simulink model "Problem3_sim"  (R2018a)
settings: Solver=ode45  StartTime=0.0  StopTime=600  RelTol=1e-3
values from neighbouring files (symbols this model uses):
  g = 9.81    [Problem3.m]
  kd_fi = (2*zeta_fi*omega_fi-alpha_fi1)/alpha_fi2    [Problem3.m]
  ki_chi = omega_chi^2*V_g/g    [Problem3.m]
  ki_fi = -0    (= 0)    [Problem3.m]
  kp_chi = 2*zeta_chi*omega_chi*V_g/g    [Problem3.m]
  kp_fi = -2    [Problem3.m]
  V_g = 580/3.6    (= 161.111111111)    [Problem3.m]
undefined symbols (not defined in the file or in its folder): data
libraries: simulink_extras x2
settings Model: Creator=marti  LastModifiedBy=Anders Vagle
settings OptimizationCC: LifeSpan=inf
settings DebuggingCC: SFExecutionAtInitializationDiag=none
settings HardwareCC: ProdBitPerSizeT=32  ProdBitPerPtrDiffT=32  ProdWordSize=32  ProdHWDeviceType=Specified
settings CodeAppCC: StateflowObjectComments=on

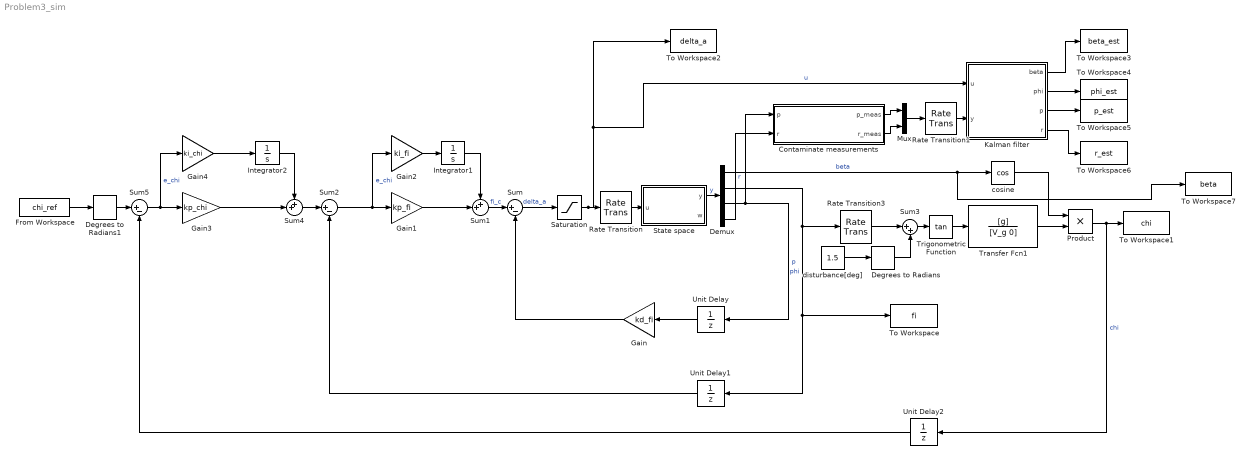
== system Problem3_sim ==
  Contaminate measurements : MATLAB Function  TreatAsAtomicUnit=on
  Degrees to Radians : simulink_extras/Transformations/Degrees to Radians
  Degrees to Radians1 : simulink_extras/Transformations/Degrees to Radians
  Demux : Demux
  From Workspace : FromWorkspace  VariableName=chi_ref  SampleTime=0  Interpolate=off  OutputAfterFinalValue=Holding final value
  Gain : Gain  Gain=kd_fi
  Gain1 : Gain  Gain=kp_fi
  Gain2 : Gain  Gain=ki_fi
  Gain3 : Gain  Gain=kp_chi
  Gain4 : Gain  Gain=ki_chi
  Integrator1 : Integrator
  Integrator2 : Integrator
  Kalman filter : MATLAB Function  TreatAsAtomicUnit=on  mask{data=data}
      mask prompts: data "data struct"
  Mux : Mux  Inputs=2
  Product : Product
  Rate Transition : RateTransition  OutPortSampleTime=Ts
  Rate Transition1 : RateTransition
  Rate Transition3 : RateTransition  OutPortSampleTime=Ts
  Saturation : Saturate  UpperLimit=30/180*pi  LowerLimit=-30/180*pi
  State space : MATLAB Function  TreatAsAtomicUnit=on
  Sum : Sum  Inputs=|+-
  Sum1 : Sum  Inputs=++|
  Sum2 : Sum  Inputs=|+-
  Sum3 : Sum  Inputs=|++
  Sum4 : Sum  Inputs=++|
  Sum5 : Sum  Inputs=|+-
  To Workspace : ToWorkspace  VariableName=fi  SaveFormat=Timeseries  SampleTime=-1
  To Workspace1 : ToWorkspace  VariableName=chi  SaveFormat=Timeseries  SampleTime=-1
  To Workspace2 : ToWorkspace  VariableName=delta_a  SaveFormat=Timeseries  SampleTime=-1
  To Workspace3 : ToWorkspace  VariableName=beta_est  SaveFormat=Timeseries  SampleTime=-1
  To Workspace4 : ToWorkspace  VariableName=phi_est  SaveFormat=Timeseries  SampleTime=-1
  To Workspace5 : ToWorkspace  VariableName=p_est  SaveFormat=Timeseries  SampleTime=-1
  To Workspace6 : ToWorkspace  VariableName=r_est  SaveFormat=Timeseries  SampleTime=-1
  To Workspace7 : ToWorkspace  VariableName=beta  SaveFormat=Timeseries  SampleTime=-1
  Transfer Fcn1 : TransferFcn  Numerator=[g]  Denominator=[V_g 0]
  Trigonometric Function : Trigonometry  Operator=tan
  Unit Delay : UnitDelay  SampleTime=-1
  Unit Delay1 : UnitDelay  SampleTime=-1
  Unit Delay2 : UnitDelay  SampleTime=-1
  cosine : Trigonometry  Operator=cos
  disturbance[deg] : Constant  Value=1.5
  wires:
  Gain/1 -> Sum/2
  Sum1/1 -> Sum/1  "fi_c"
  Integrator1/1 -> Sum1/1
  Gain1/1 -> Sum1/2
  Sum2/1 -> Gain2/1, Gain1/1  "e_chi"
  Demux/2 -> Rate Transition3/1, Unit Delay1/1, To Workspace/1  "phi"
  Integrator2/1 -> Sum4/1
  Gain3/1 -> Sum4/2
  Sum5/1 -> Gain4/1, Gain3/1  "e_chi"
  Sum/1 -> Saturation/1  "delta_a"
  Sum4/1 -> Sum2/1
  Degrees to Radians1/1 -> Sum5/1
  disturbance[deg]/1 -> Degrees to Radians/1
  From Workspace/1 -> Degrees to Radians1/1
  Sum3/1 -> Trigonometric Function/1
  Trigonometric Function/1 -> Transfer Fcn1/1
  Demux/1 -> To Workspace7/1, cosine/1  "beta"
  Transfer Fcn1/1 -> Product/2
  Product/1 -> Unit Delay2/1, To Workspace1/1  "chi"
  Saturation/1 -> To Workspace2/1, Kalman filter/1(u), Rate Transition/1  "u"
  State space/1(y) -> Demux/1  "y"
  Demux/3 -> Contaminate measurements/1(p), Unit Delay/1  "p"
  Gain2/1 -> Integrator1/1
  Gain4/1 -> Integrator2/1
  Degrees to Radians/1 -> Sum3/2
  Demux/4 -> Contaminate measurements/2(r)  "r"
  Contaminate measurements/2(r_meas) -> Mux/2
  Contaminate measurements/1(p_meas) -> Mux/1
  Kalman filter/1(beta) -> To Workspace3/1
  Kalman filter/2(phi) -> To Workspace4/1
  Kalman filter/3(p) -> To Workspace5/1
  Kalman filter/4(r) -> To Workspace6/1
  Rate Transition/1 -> State space/1(u)
  Unit Delay/1 -> Gain/1
  Unit Delay1/1 -> Sum2/2
  Mux/1 -> Rate Transition1/1
  Rate Transition1/1 -> Kalman filter/2(y)
  cosine/1 -> Product/1
  Unit Delay2/1 -> Sum5/2
  Rate Transition3/1 -> Sum3/1

== matlab function Problem3_sim/Contaminate measurements ==
  data: p input; p_meas output; r input; r_meas output
function [p_meas, r_meas] = contaminate(p, r)

% persistent counter; % Variable for checking if it is the first iteration.
% coder.extrinsic('randn','rng');
% if isempty(counter)
%    counter = 1;
%    rng('shuffle'); % Necessary for generating unique process noise for every simulation.
% end

% var_p = 0.2^2;
% var_r = 0.2^2;

p_meas = p + randn(1,1)*sqrt(0.2^2);
r_meas = r + randn(1,1)*sqrt(0.2^2);

== matlab function Problem3_sim/State space ==
  data: u input; y output; w output
function [y, w] = state_space(u)
% Generate the output of the state space

    % Persistent variables to be kept between function calls
    persistent counter; % Variable for checking if it is the first iteration.
    persistent x;       % The state x
    
   % The next line is necessary for generating unique process noise for every simulation.
   % Otherwise, the noise will be equal every time you run the simulation,
   % even though it is white. This has to do with how Matlab generates
   % random numbers. 
   coder.extrinsic('randn','rng');
    
    h = 0.01;       % Time step of Euler integration
    delta_a_c = u;  % Aileron input
    
    if isempty(counter)
      % First iteration
        counter = 1;
           
        % Initialize state space
        x = zeros(5,1);
        w = zeros(5,1); 
        rng('shuffle'); % Necessary for generating unique process noise for every simulation.
    
    else
        % State-space matrices
        A = [-0.322, 0.052, 0.028, -1.12, 0.002;
             0, 0, 1, -0.001, 0;
             -10.6, 0, -2.87, 0.46, -0.65;
             6.87, 0, -0.04, -0.32, -0.02;
             0, 0, 0, 0, -7.5];
 
        B = [0; 0; 0; 0; 7.5;];
        
        E = eye(5);
        
        % Discrete version
        Ad = eye(5) + h*A;
        Bd = h*B;
        Ed = E;
        
        % The Qd matrix in the assignment is given directly in discrete-time here and
        % therefore, it is not necessary to discretize E.
        Qd = h*10^-6*[0.001, 0, 0, 0, 0;
                  0, 1, 0, 0, 0;
                  0, 0, 100, 0, 0;
                  0, 0, 0, 10, 0;
                  0, 0, 0, 0, 0];
          
        w = sqrt(Qd)*randn(5,1,1); % The standard deviation must be multiplied with random numbers with a zero-mean unit variance random number to generate process noise. 
        
        % Discrete-time state space update
        x = Ad*x + Bd * delta_a_c + Ed*w;
    end
    y = x(1:4); % Return every state except the actuator state.
end

== matlab function Problem3_sim/Kalman filter ==
  settings: updateMethod=DISCRETE  sampleTime=Ts
  data: beta output; u input; y input; data parameter; phi output; p output; r output
function [beta,phi,p,r]  = Kalman_filter(u,y,data)
persistent xpri xhat P;

A = data.A;
B = data.B;
C = data.C;
Q = data.Q;
R = data.R;
I = data.I;
if isempty(xpri)
    xpri = data.xhat0;
    P = data.P;
end

K = P*C'/(C*P*C' + R);
xhat = xpri + K*(y - C*xpri);
P = (I - K*C)*P*(I - K*C)' + K*R*K';

xpri = A*xhat + B*u;
P = A*P*A' + Q;

beta = xhat(1);
phi = xhat(2);
p = xhat(3);
r = xhat(4);
